simulink model "matlab_function"  (R2012b)
settings: Solver=ode45  StartTime=0.0  StopTime=1  MaxStep=0.1  RelTol=1e-3
libraries: simulink x5
settings Model: Creator=Kushal  LastModifiedBy=Kushal

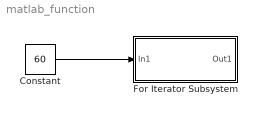
== system matlab_function ==
  Constant : Constant  Value=60
  For Iterator Subsystem : Subsystem  TreatAsAtomicUnit=on
  wires:
  Constant/1 -> For Iterator Subsystem/1(In1)

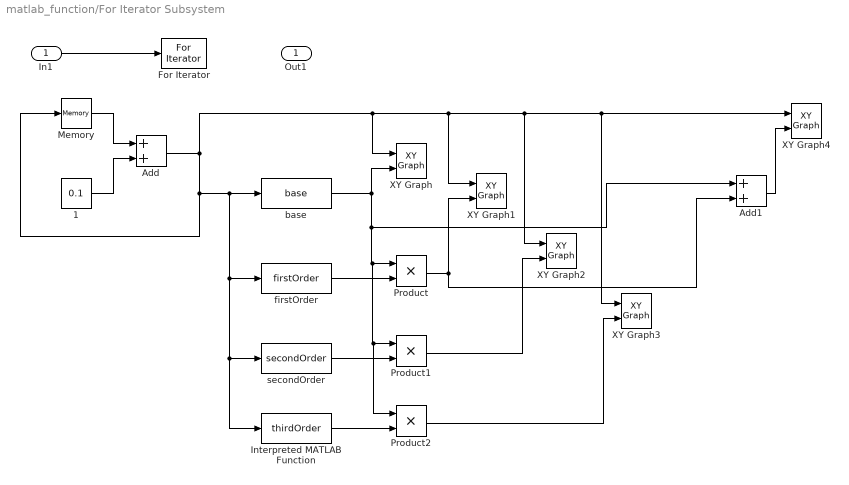
== system matlab_function/For Iterator Subsystem ==
  In1 : Inport
  1 : Constant  Value=0.1
  Add : Sum
  Add1 : Sum
  For Iterator : ForIterator  ResetStates=reset  IterationSource=external
  Interpreted MATLAB Function : MATLABFcn  MATLABFcn=thirdOrder
  Memory : Memory  X0=-3.1  InheritSampleTime=on
  Product : Product  RndMeth=Zero
  Product1 : Product  RndMeth=Zero
  Product2 : Product  RndMeth=Zero
  XY Graph : simulink/Sinks/XY Graph  xmin=-3  xmax=3  ymin=0  ymax=1  st=-1
  XY Graph1 : simulink/Sinks/XY Graph  xmin=-3  xmax=3  ymin=-1.6  ymax=1.6  st=-1
  XY Graph2 : simulink/Sinks/XY Graph  xmin=-3  xmax=3  ymin=-6.5  ymax=3  st=-1
  XY Graph3 : simulink/Sinks/XY Graph  xmin=-3  xmax=3  ymin=-22  ymax=22  st=-1
  XY Graph4 : simulink/Sinks/XY Graph  xmin=-3  xmax=3  ymin=-22  ymax=22  st=-1
  base : MATLABFcn  MATLABFcn=base
  firstOrder : MATLABFcn  MATLABFcn=firstOrder
  secondOrder : MATLABFcn  MATLABFcn=secondOrder
  Out1 : Outport
  wires:
  In1/1 -> For Iterator/1
  Memory/1 -> Add/1
  1/1 -> Add/2
  Product/1 -> XY Graph1/2, Add1/2
  firstOrder/1 -> Product/2
  secondOrder/1 -> Product1/2
  Product1/1 -> XY Graph2/2
  Interpreted MATLAB Function/1 -> Product2/2
  Product2/1 -> XY Graph3/2
  Add/1 -> Memory/1, firstOrder/1, Interpreted MATLAB Function/1, secondOrder/1, base/1, XY Graph/1, XY Graph3/1, XY Graph4/1, XY Graph2/1, XY Graph1/1
  base/1 -> Add1/1, Product2/1, Product1/1, Product/1, XY Graph/2
  Add1/1 -> XY Graph4/2
